simulink model "Clik_Jacobian_transpose"  (R2023b)
settings: Solver=VariableStepAuto  StartTime=0.0  StopTime=20  RelTol=1e-3
model workspace: external: MAT-File (data not in the file)
undefined symbols (not defined in the file): DiscIntNeverNeededParam, f_s
settings Model: Creator=benit  LastModifiedBy=ANDREA
settings OptimizationCC: ReuseModelBlockBuffer=off

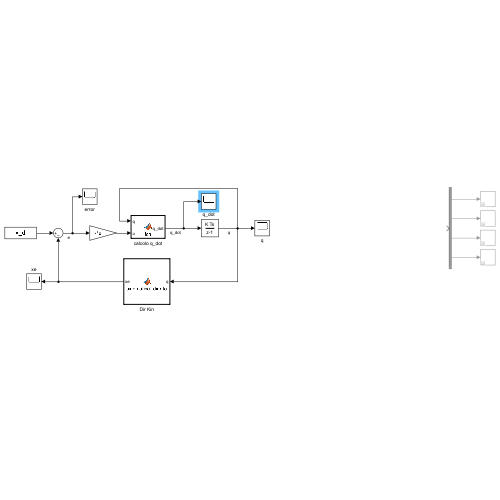
[thumbnail: Simulink's stored preview of the top-level diagram]
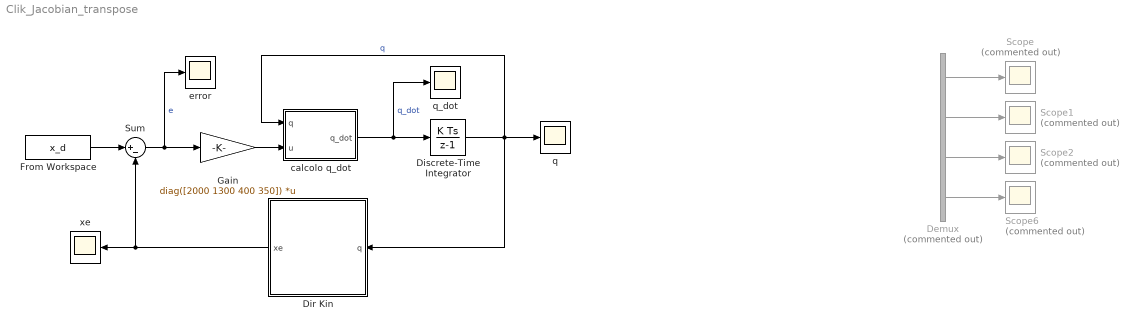
== system Clik_Jacobian_transpose ==
  Demux : Demux  Commented=on
  Dir Kin : MATLAB Function  TreatAsAtomicUnit=on
  Discrete-Time Integrator : DiscreteIntegrator  gainval=1  InitialCondition=config_p_init'  SampleTime=1/f_s  ICPrevOutput=DiscIntNeverNeededParam  ICPrevScaledInput=DiscIntNeverNeededParam
  From Workspace : FromWorkspace  VariableName=x_d
  Gain : Gain  Gain=diag([2000 1300 400 350])  Multiplication=Matrix(K*u)
  Scope{,1..2,6} (4 alike) : Scope  Commented=on
  Sum : Sum  Inputs=|+-
  calcolo q_dot : MATLAB Function  TreatAsAtomicUnit=on
  error : Scope
  q : Scope
  q_dot : Scope
  xe : Scope
  wires:
  Sum/1 -> error/1, Gain/1  "e"
  Demux/1 -> Scope/1
  Demux/2 -> Scope1/1
  Demux/3 -> Scope2/1
  From Workspace/1 -> Sum/1
  Discrete-Time Integrator/1 -> q/1, calcolo q_dot/1(q), Dir Kin/1(q)  "q"
  calcolo q_dot/1(q_dot) -> q_dot/1, Discrete-Time Integrator/1  "q_dot"
  Dir Kin/1(xe) -> xe/1, Sum/2
  Gain/1 -> calcolo q_dot/2(u)
  Demux/4 -> Scope6/1

== matlab function Clik_Jacobian_transpose/calcolo q_dot ==
  data: q input; u input; q_dot output
function q_dot = fcn(q,u)

    J = [-0.5*sin(q(1))-0.5*sin(q(1)+q(2))   -0.5*sin(q(1)+q(2))    0  0 
          0.5*cos(q(1))+0.5*cos(q(1)+q(2))    0.5*cos(q(1)+q(2))    0  0 
          0                                   0                    -1  0
          1                                   1                     0  -1];
    
    q_dot = J'*u;

end

== matlab function Clik_Jacobian_transpose/Dir Kin ==
  data: q input; xe output
function xe = cinematica_diretta(q)
    
    xe = [  0.5*cos(q(1))+0.5*cos(q(1)+q(2));
            0.5*sin(q(1))+0.5*sin(q(1)+q(2));
            1/2-q(3)
            q(1)+q(2)-q(4) ];

end
